simulink model "Counter3bits"  (R2025b)
settings: Solver=VariableStepAuto  StartTime=0.0  StopTime=Inf  RelTol=1e-3
settings Model: Creator=Soochan Kim  LastModifiedBy=Soochan Kim

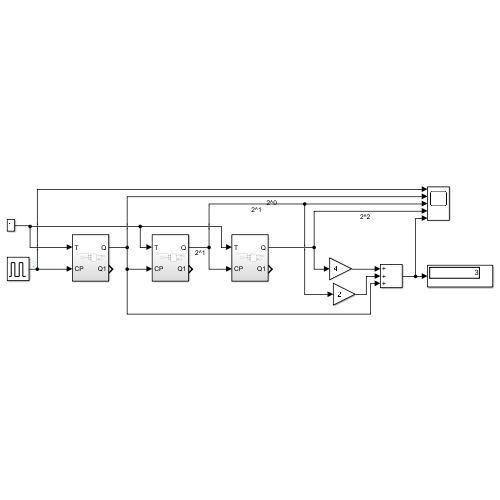
[thumbnail: Simulink's stored preview of the top-level diagram]
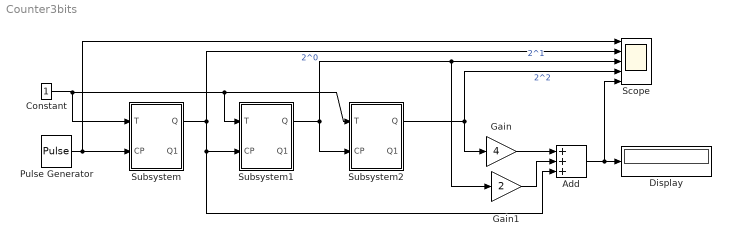
== system Counter3bits ==
  Add : Sum  Inputs=+++
  Constant : Constant
  Display : Display
  Gain : Gain  Gain=4
  Gain1 : Gain  Gain=2
  Pulse Generator : DiscretePulseGenerator  PulseType=Time based  Period=1  PulseWidth=50  PhaseDelay=0.5
  Scope : Scope  NumInputPorts=5
      settings: ActiveDisplayYMinimum=-0.12499999999999997  ActiveDisplayYMaximum=1.125
  Subsystem : Subsystem
  Subsystem1 : Subsystem
  Subsystem2 : Subsystem
  wires:
  Pulse Generator/1 -> Subsystem/2(CP), Scope/1
  Subsystem1/1(Q) -> Subsystem2/2(CP), Gain1/1, Scope/3  "2^1"
  Subsystem2/1(Q) -> Gain/1, Scope/4  "2^2"
  Subsystem/1(Q) -> Subsystem1/2(CP), Add/3, Scope/2  "2^0"
  Constant/1 -> Subsystem1/1(T), Subsystem2/1(T), Subsystem/1(T)
  Gain/1 -> Add/1
  Add/1 -> Scope/5, Display/1
  Gain1/1 -> Add/2

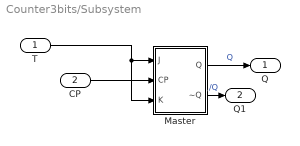
== system Counter3bits/Subsystem ==
  T : Inport
  CP : Inport  Port=2
  Master : Subsystem
  Q : Outport
  Q1 : Outport  Port=2
  wires:
  T/1 -> Master/3(K), Master/1(J)
  CP/1 -> Master/2(CP)
  Master/2(~Q) -> Q1/1  "/Q"
  Master/1(Q) -> Q/1  "Q"

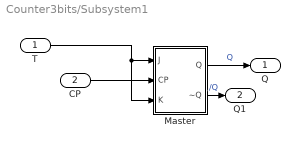
== system Counter3bits/Subsystem1 ==
  T : Inport
  CP : Inport  Port=2
  Master : Subsystem
  Q : Outport
  Q1 : Outport  Port=2
  wires:
  T/1 -> Master/3(K), Master/1(J)
  CP/1 -> Master/2(CP)
  Master/2(~Q) -> Q1/1  "/Q"
  Master/1(Q) -> Q/1  "Q"

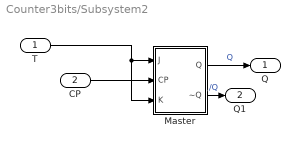
== system Counter3bits/Subsystem2 ==
  T : Inport
  CP : Inport  Port=2
  Master : Subsystem
  Q : Outport
  Q1 : Outport  Port=2
  wires:
  T/1 -> Master/3(K), Master/1(J)
  CP/1 -> Master/2(CP)
  Master/2(~Q) -> Q1/1  "/Q"
  Master/1(Q) -> Q/1  "Q"

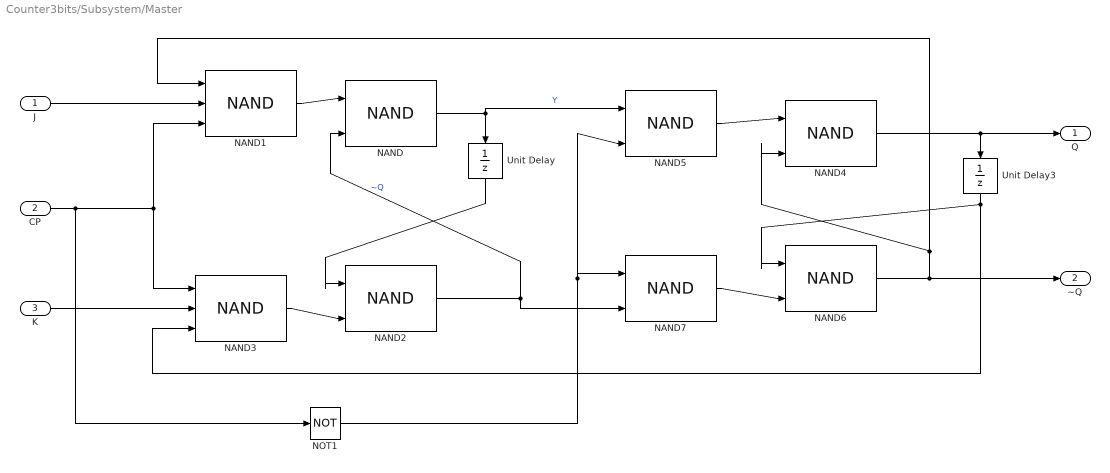
== system Counter3bits/Subsystem/Master ==
  J : Inport
  CP : Inport  Port=2
  K : Inport  Port=3
  NAND{,2,4..7} (6 alike) : Logic  Operator=NAND  IconShape=distinctive  AllPortsSameDT=off  OutDataTypeStr=boolean
  NAND1 : Logic  Operator=NAND  Inputs=3  IconShape=distinctive  AllPortsSameDT=off  OutDataTypeStr=boolean
  NAND3 : Logic  Operator=NAND  Inputs=3  IconShape=distinctive  AllPortsSameDT=off  OutDataTypeStr=boolean
  NOT1 : Logic  Operator=NOT  IconShape=distinctive  AllPortsSameDT=off  OutDataTypeStr=boolean
  Unit Delay : UnitDelay  SampleTime=0.001  HasFrameUpgradeWarning=on
  Unit Delay3 : UnitDelay  SampleTime=-1  HasFrameUpgradeWarning=on
  Q : Outport
  ~Q : Outport  Port=2
  wires:
  NAND/1 -> Unit Delay/1, NAND5/1  "Y"
  NAND2/1 -> NAND/2, NAND7/2  "~Q"
  Unit Delay/1 -> NAND2/1
  K/1 -> NAND3/2
  NAND1/1 -> NAND/1
  NAND3/1 -> NAND2/2
  J/1 -> NAND1/2
  NAND6/1 -> ~Q/1, NAND1/1, NAND4/2
  Unit Delay3/1 -> NAND3/3, NAND6/1
  NAND5/1 -> NAND4/1
  NAND7/1 -> NAND6/2
  NAND4/1 -> Q/1, Unit Delay3/1
  CP/1 -> NAND1/3, NAND3/1, NOT1/1
  NOT1/1 -> NAND5/2, NAND7/1

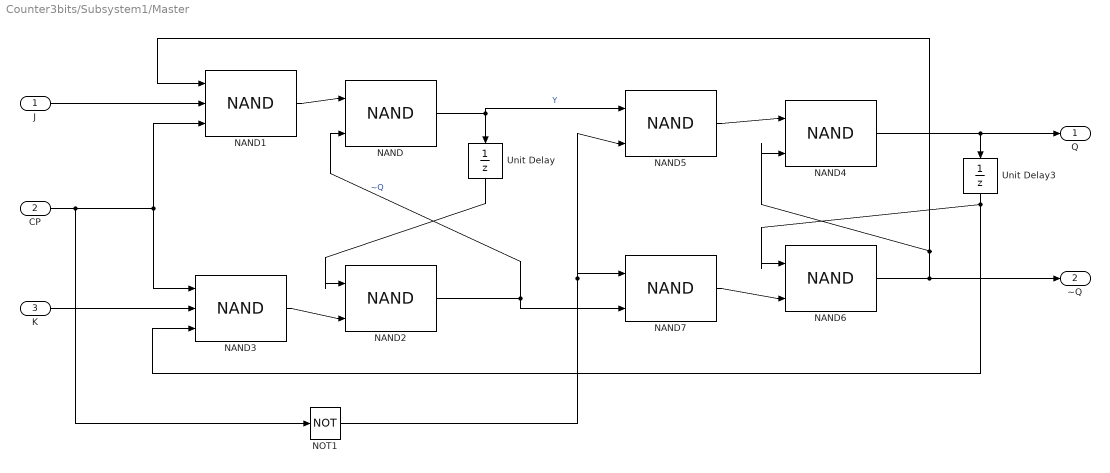
== system Counter3bits/Subsystem1/Master ==
  J : Inport
  CP : Inport  Port=2
  K : Inport  Port=3
  NAND{,2,4..7} (6 alike) : Logic  Operator=NAND  IconShape=distinctive  AllPortsSameDT=off  OutDataTypeStr=boolean
  NAND1 : Logic  Operator=NAND  Inputs=3  IconShape=distinctive  AllPortsSameDT=off  OutDataTypeStr=boolean
  NAND3 : Logic  Operator=NAND  Inputs=3  IconShape=distinctive  AllPortsSameDT=off  OutDataTypeStr=boolean
  NOT1 : Logic  Operator=NOT  IconShape=distinctive  AllPortsSameDT=off  OutDataTypeStr=boolean
  Unit Delay : UnitDelay  SampleTime=0.001  HasFrameUpgradeWarning=on
  Unit Delay3 : UnitDelay  SampleTime=-1  HasFrameUpgradeWarning=on
  Q : Outport
  ~Q : Outport  Port=2
  wires:
  NAND/1 -> Unit Delay/1, NAND5/1  "Y"
  NAND2/1 -> NAND/2, NAND7/2  "~Q"
  Unit Delay/1 -> NAND2/1
  K/1 -> NAND3/2
  NAND1/1 -> NAND/1
  NAND3/1 -> NAND2/2
  J/1 -> NAND1/2
  NAND6/1 -> ~Q/1, NAND1/1, NAND4/2
  Unit Delay3/1 -> NAND3/3, NAND6/1
  NAND5/1 -> NAND4/1
  NAND7/1 -> NAND6/2
  NAND4/1 -> Q/1, Unit Delay3/1
  CP/1 -> NAND1/3, NAND3/1, NOT1/1
  NOT1/1 -> NAND5/2, NAND7/1

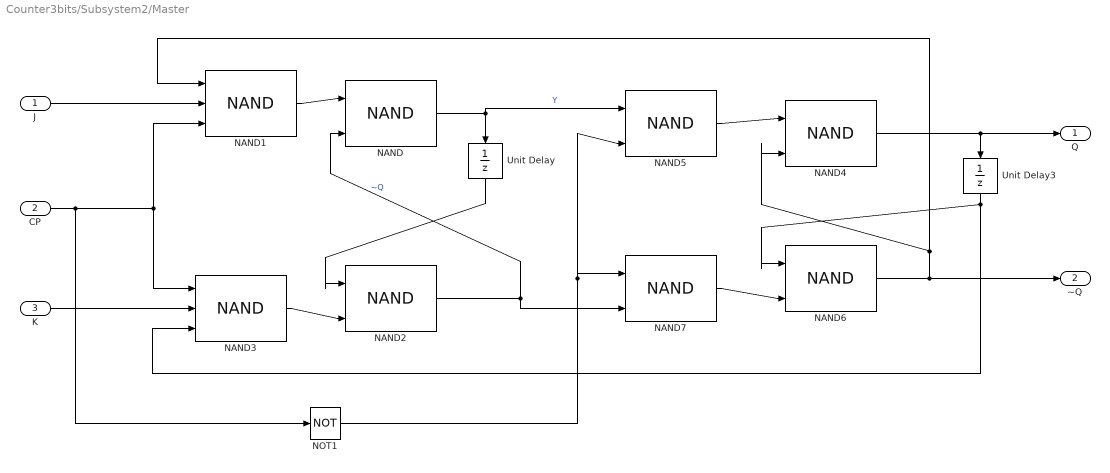
== system Counter3bits/Subsystem2/Master ==
  J : Inport
  CP : Inport  Port=2
  K : Inport  Port=3
  NAND{,2,4..7} (6 alike) : Logic  Operator=NAND  IconShape=distinctive  AllPortsSameDT=off  OutDataTypeStr=boolean
  NAND1 : Logic  Operator=NAND  Inputs=3  IconShape=distinctive  AllPortsSameDT=off  OutDataTypeStr=boolean
  NAND3 : Logic  Operator=NAND  Inputs=3  IconShape=distinctive  AllPortsSameDT=off  OutDataTypeStr=boolean
  NOT1 : Logic  Operator=NOT  IconShape=distinctive  AllPortsSameDT=off  OutDataTypeStr=boolean
  Unit Delay : UnitDelay  SampleTime=0.001  HasFrameUpgradeWarning=on
  Unit Delay3 : UnitDelay  SampleTime=-1  HasFrameUpgradeWarning=on
  Q : Outport
  ~Q : Outport  Port=2
  wires:
  NAND/1 -> Unit Delay/1, NAND5/1  "Y"
  NAND2/1 -> NAND/2, NAND7/2  "~Q"
  Unit Delay/1 -> NAND2/1
  K/1 -> NAND3/2
  NAND1/1 -> NAND/1
  NAND3/1 -> NAND2/2
  J/1 -> NAND1/2
  NAND6/1 -> ~Q/1, NAND1/1, NAND4/2
  Unit Delay3/1 -> NAND3/3, NAND6/1
  NAND5/1 -> NAND4/1
  NAND7/1 -> NAND6/2
  NAND4/1 -> Q/1, Unit Delay3/1
  CP/1 -> NAND1/3, NAND3/1, NOT1/1
  NOT1/1 -> NAND5/2, NAND7/1
